simulink model "ex1"  (R2024a)
settings: Solver=VariableStepAuto  StartTime=0.0  StopTime=20.0  RelTol=1e-6
undefined symbols (not defined in the file or in its folder): A, B, Bf, Cz, Dz, G, K1, K2, w_0, x_0
settings Model: Creator=admin  LastModifiedBy=anton
settings RTWCC: GPUComputeCapability=3.5

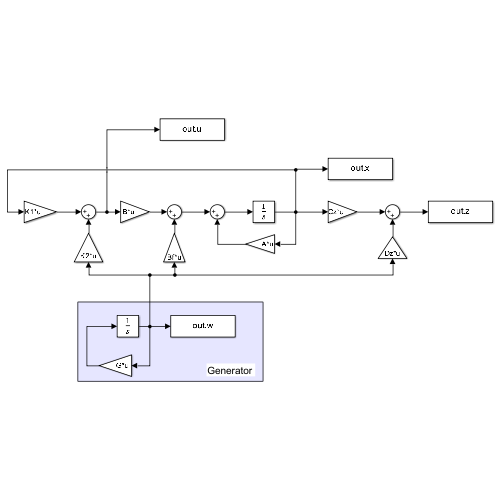
[thumbnail: Simulink's stored preview of the top-level diagram]
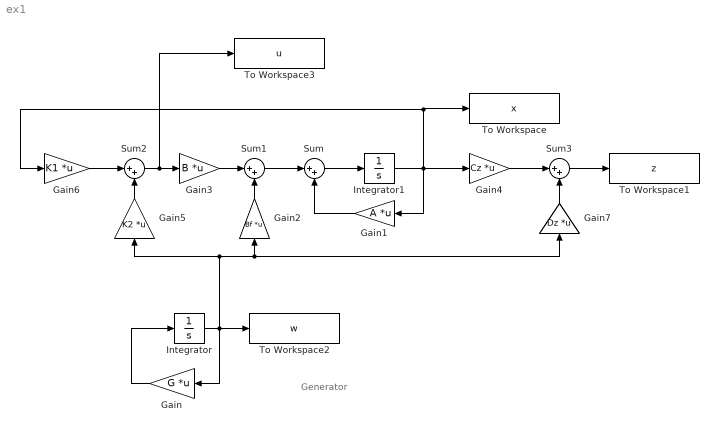
== system ex1 ==
  note: Generator
  Gain : Gain  Gain=G  Multiplication=Matrix(K*u)
  Gain1 : Gain  Gain=A  Multiplication=Matrix(K*u)
  Gain2 : Gain  Gain=Bf  Multiplication=Matrix(K*u)
  Gain3 : Gain  Gain=B  Multiplication=Matrix(K*u)
  Gain4 : Gain  Gain=Cz  Multiplication=Matrix(K*u)
  Gain5 : Gain  Gain=K2  Multiplication=Matrix(K*u)
  Gain6 : Gain  Gain=K1  Multiplication=Matrix(K*u)
  Gain7 : Gain  Gain=Dz  Multiplication=Matrix(K*u)
  Integrator : Integrator  InitialCondition=w_0
  Integrator1 : Integrator  InitialCondition=x_0
  Sum{,1..3} (4 alike) : Sum  Inputs=|++
  To Workspace : ToWorkspace  VariableName=x  SaveFormat=Timeseries  SampleTime=-1
  To Workspace1 : ToWorkspace  VariableName=z  SaveFormat=Timeseries  SampleTime=-1
  To Workspace2 : ToWorkspace  VariableName=w  SaveFormat=Timeseries  SampleTime=-1
  To Workspace3 : ToWorkspace  VariableName=u  SaveFormat=Timeseries  SampleTime=-1
  wires:
  Integrator/1 -> Gain2/1, Gain7/1, Gain5/1, To Workspace2/1, Gain/1
  Sum/1 -> Integrator1/1
  Gain1/1 -> Sum/2
  Integrator1/1 -> Gain1/1, To Workspace/1, Gain6/1, Gain4/1
  Sum1/1 -> Sum/1
  Gain2/1 -> Sum1/2
  Gain/1 -> Integrator/1
  Gain3/1 -> Sum1/1
  Sum2/1 -> To Workspace3/1, Gain3/1
  Gain5/1 -> Sum2/2
  Gain6/1 -> Sum2/1
  Gain4/1 -> Sum3/1
  Sum3/1 -> To Workspace1/1
  Gain7/1 -> Sum3/2
